simulink model "lab4"  (R2018a)
settings: Solver=VariableStepAuto  StartTime=0.0  StopTime=800  RelTol=1e-3
libraries: simulink x1
settings Model: Creator=Luka  LastModifiedBy=Luka

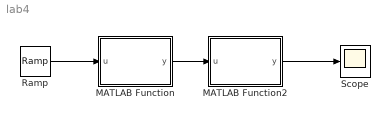
== system lab4 ==
  MATLAB Function : MATLAB Function  TreatAsAtomicUnit=on
  MATLAB Function2 : MATLAB Function  TreatAsAtomicUnit=on
  Ramp : simulink/Sources/Ramp  slope=1  start=0  InitialOutput=0
  Scope : Scope
  wires:
  MATLAB Function2/1(y) -> Scope/1
  MATLAB Function/1(y) -> MATLAB Function2/1(u)
  Ramp/1 -> MATLAB Function/1(u)

== matlab function lab4/MATLAB Function ==
  data: u input; y output
function y = fcn(u)

y = 50*(1-exp(-0.005*u));

== matlab function lab4/MATLAB Function2 ==
  data: u input; y output
function y = fcn(u)

y = -200*log(1 - u/50);
